simulink model "simulation_maglev_control"  (R2023a)
settings: Solver=VariableStepAuto  StartTime=0.0  StopTime=10  MaxStep=0.001  RelTol=1e-3
settings Model: Creator=91936  LastModifiedBy=91936
settings RTWCC: GPUComputeCapability=5.0
settings ConfigComp: CovBoundaryAbsTol=1.0e-5

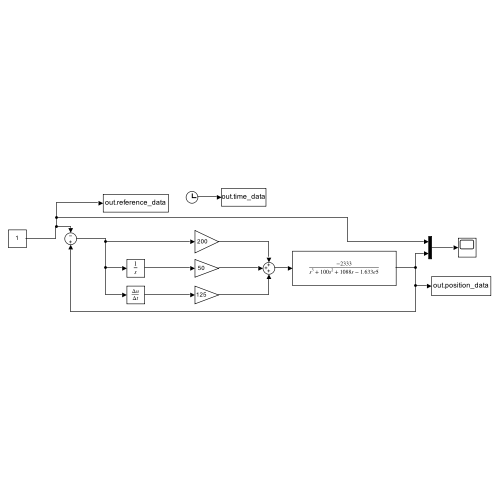
[thumbnail: Simulink's stored preview of the top-level diagram]
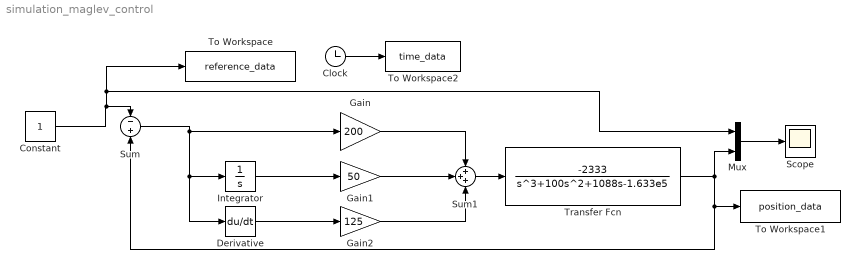
== system simulation_maglev_control ==
  Clock : Clock
  Constant : Constant
  Derivative : Derivative
  Gain : Gain  Gain=200
  Gain1 : Gain  Gain=50
  Gain2 : Gain  Gain=125
  Integrator : Integrator
  Mux : Mux  Inputs=2
  Scope : Scope
  Sum : Sum  Inputs=-+
  Sum1 : Sum  Inputs=+++
  To Workspace : ToWorkspace  VariableName=reference_data  SampleTime=-1
  To Workspace1 : ToWorkspace  VariableName=position_data  SampleTime=-1
  To Workspace2 : ToWorkspace  VariableName=time_data  SampleTime=-1
  Transfer Fcn : TransferFcn  Numerator=[-2333]  Denominator=[1 100 1088 -1.633e5]
  wires:
  Constant/1 -> To Workspace/1, Mux/1, Sum/1
  Integrator/1 -> Gain1/1
  Derivative/1 -> Gain2/1
  Gain/1 -> Sum1/1
  Gain1/1 -> Sum1/2
  Gain2/1 -> Sum1/3
  Sum1/1 -> Transfer Fcn/1
  Transfer Fcn/1 -> Sum/2, To Workspace1/1, Mux/2
  Mux/1 -> Scope/1
  Clock/1 -> To Workspace2/1
  Sum/1 -> Derivative/1, Integrator/1, Gain/1
